simulink model "ep4_3"  (R2018a)
settings: Solver=ode45  StartTime=0.0  StopTime=10.0  MaxStep=0.005  RelTol=1e-3
settings Model: Creator=zheny  LastModifiedBy=zheny

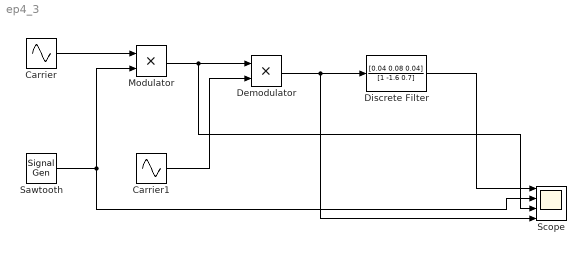
== system ep4_3 ==
  Carrier : Sin  Frequency=1000  SampleTime=0
  Carrier1 : Sin  Frequency=1000  SampleTime=0.005
  Demodulator : Product
  Discrete Filter : DiscreteFilter  Numerator=[0.04 0.08 0.04]  Denominator=[1 -1.6 0.7]  SampleTime=0.005
  Modulator : Product
  Sawtooth : SignalGenerator  WaveForm=sawtooth
  Scope : Scope  NumInputPorts=4
  wires:
  Discrete Filter/1 -> Scope/1
  Demodulator/1 -> Scope/4, Discrete Filter/1
  Modulator/1 -> Scope/3, Demodulator/1
  Carrier/1 -> Modulator/1
  Carrier1/1 -> Demodulator/2
  Sawtooth/1 -> Scope/2, Modulator/2
